simulink model "Floating_Scope"  (R2020a)
settings: Solver=VariableStepAuto  StartTime=0.0  StopTime=10.0  RelTol=1e-3
settings Model: Creator=royde  LastModifiedBy=royde

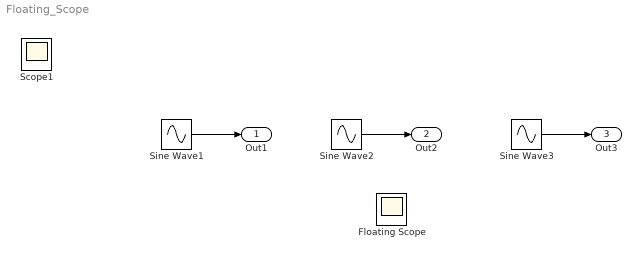
== system Floating_Scope ==
  Floating Scope : Scope
      settings: Floating=on
  Sine Wave1 : Sin  SampleTime=0
  Sine Wave2 : Sin  Amplitude=2  SampleTime=0
  Sine Wave3 : Sin  Amplitude=3  SampleTime=0
  Out1 : Outport
  Out2 : Outport  Port=2
  Out3 : Outport  Port=3
  Scope1 : Scope
  wires:
  Sine Wave1/1 -> Out1/1
  Sine Wave2/1 -> Out2/1
  Sine Wave3/1 -> Out3/1
